simulink model "beisp_3"  (Simulink 4.00)
settings: Solver=ode5  SolverMode=SingleTasking  StartTime=0.0  StopTime=10.0  RelTol=1e-3  AbsTol=1e-6
settings Model: LastModifiedBy=Administrator  LoadExternalInput=on  ExternalInput=A1  LimitDataPoints=off  RTWOptions="-aExtMode=0 -aForceParamTrailComments=0 -aInlineInvariantSignals=0 -aLocalBlockOutputs=1 -aLogVarNameModifier=\"rt_\" -aRTWVerbose=1 -aRollThreshold=5 -aShowEliminatedStatements=1"  ExtModeTrigMode=oneshot  ExtModeArmWhenConnect=off  BlockReductionOpt=off

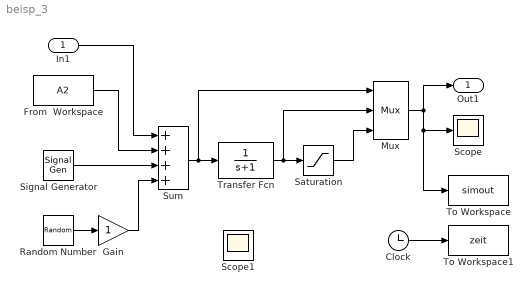
== system beisp_3 ==
  In1 : Inport  Port=1
  Clock : Clock
      settings: DisplayTime=off  Decimation=10
  From  Workspace : FromWorkspace  VariableName=A2  SampleTime=0  OutputAfterFinalValue=Extrapolation
  Gain : Gain  Gain=1  Multiplication=Element-wise(K.*u)  SaturateOnIntegerOverflow=on
  Mux : Mux  Inputs=3
      settings: DisplayOption=none
  Random Number : RandomNumber  Mean=0  Variance=1  Seed=0  SampleTime=0
  Saturation : Saturate  UpperLimit=4.5  LowerLimit=-4.5  LinearizeAsGain=on
  Scope : Scope
      settings: TickLabels=on  TimeRange=auto  YMin=-5  YMax=5  SaveToWorkspace=off  SaveName=ScopeData  DataFormat=Array  LimitDataPoints=on  MaxDataPoints=5000
  Scope1 : Scope
      settings: Floating=on  TickLabels=on  TimeRange=auto  YMin=-5  YMax=5  SaveToWorkspace=off  SaveName=ScopeData  DataFormat=Array  LimitDataPoints=on  MaxDataPoints=5000
  Signal Generator : SignalGenerator  WaveForm=square  Amplitude=5  Frequency=0.15  Units=Hertz
  Sum : Sum  Inputs=++++  SaturateOnIntegerOverflow=on
  To Workspace : ToWorkspace  VariableName=simout  SampleTime=-1  SaveFormat=Array
      settings: MaxDataPoints=1000
  To Workspace1 : ToWorkspace  VariableName=zeit  SampleTime=-1  SaveFormat=Array
      settings: MaxDataPoints=1000
  Transfer Fcn : TransferFcn  Numerator=[1]  Denominator=[1 1]  Realization=auto  AbsoluteTolerance=auto
  Out1 : Outport  Port=1
  wires:
  Signal Generator/1 -> Sum/3
  From  Workspace/1 -> Sum/2
  Random Number/1 -> Gain/1
  Gain/1 -> Sum/4
  Saturation/1 -> Mux/3
  Sum/1 -> Transfer Fcn/1, Mux/1
  Transfer Fcn/1 -> Saturation/1, Mux/2
  Mux/1 -> Out1/1, To Workspace/1, Scope/1
  Clock/1 -> To Workspace1/1
  In1/1 -> Sum/1
